simulink model "mBraccioSimulation"  (R2021a)
settings: Solver=VariableStepAuto  StartTime=0.0  StopTime=inf  RelTol=1e-3
undefined symbols (not defined in the file): adHomeConfig, adMotorLimits, adWaypoints, adWeight, Levenberg, Marquardt
libraries: vrlib x3, robotcorelib x2, robotmaniplib x2
settings Model: Creator=angelo  LastModifiedBy=angelo

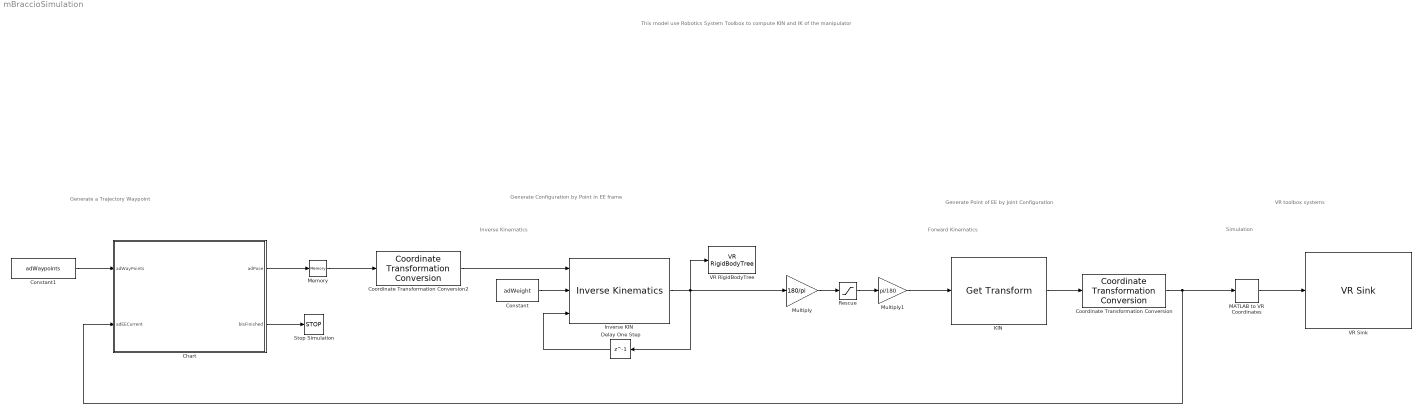
== system mBraccioSimulation ==
  note: Generate a Trajectory Waypoint
  note: Generate Point of EE by Joint Configuration
  note: Forward Kinematics
  note: Inverse Kinematics
  note: Simulation
  note: This model use Robotics System Toolbox to compute KIN and IK of the manipulator
  note: Generate Configuration by Point in EE frame
  note: VR toolbox systems
  Chart : Stateflow chart  TreatAsAtomicUnit=on
  Constant : Constant  Value=adWeight
  Constant1 : Constant  Value=adWaypoints
  Coordinate Transformation Conversion : robotcorelib/Coordinate Transformation Conversion  InputRepresentation=Homogeneous Transformation  InputEulerSequence=ZYX  ShowTrVecInputPort=on  OutputRepresentation=Translation Vector  OutputEulerSequence=ZYX  ShowTrVecOutputPort=on  SimulateUsing=Interpreted execution
      settings: SourceProductBaseCode=NV,RO,RR,UV
  Coordinate Transformation Conversion2 : robotcorelib/Coordinate Transformation Conversion  InputRepresentation=Translation Vector  InputEulerSequence=ZYX  ShowTrVecInputPort=on  OutputRepresentation=Homogeneous Transformation  OutputEulerSequence=ZYX  ShowTrVecOutputPort=on  SimulateUsing=Interpreted execution
      settings: SourceProductBaseCode=NV,RO,RR,UV
  Delay One Step : Delay  DelayLength=1  InitialCondition=adHomeConfig
  Inverse KIN : robotmaniplib/Inverse Kinematics  RigidBodyTree=oRbtBraccio  EndEffector=ee  ShowInfo=off  SolverName=Levenberg-Marquardt  EnforceJointLimits=on  MaxIterations=1500  MaxTime=10  GradientTolerance=1e-7  SolutionTolerance=1e-6  StepTolerance=1e-14  ErrorChangeTolerance=1e-12  UseErrorDamping=on  DampingBias=0.0025  SimulateUsing=Interpreted execution
  KIN : robotmaniplib/Get Transform  RigidBodyTree=oRbtBraccio  SourceBody=ee  TargetBody=base_link  SimulateUsing=Interpreted execution
  MATLAB to VR Coordinates : vrlib/Utilities/MATLAB to VR Coordinates
      settings: SourceProductBaseCode=SL
  Memory : Memory
  Multiply : Gain  Gain=180/pi
  Multiply1 : Gain  Gain=pi/180
  Rescue : Saturate  UpperLimit=adMotorLimits(:,2)  LowerLimit=adMotorLimits(:,1)
  Stop Simulation : Stop
  VR RigidBodyTree : vrlib/VR RigidBodyTree  VrmlFile=/home/angelo/1.PROJECTS/arm-manipulator-6dof/graphics/robotWorld.x3d  RBT=oRbtBraccio  useRBT=off  Ts=-1  ForceViewerOpen=off
      settings: SourceProductBaseCode=SL
  VR Sink : vrlib/VR Sink  InstantiateOnLoad=on  SampleTime=0.1  ViewEnable=on  RemoteChange=off  RemoteView=off  FieldsWritten=SetPoint.translation.3.1.1.double  WorldFileName=graphics/robotWorld.x3d  AutoView=on  VideoDimensions=[]  AllowVariableSize=off
  wires:
  Delay One Step/1 -> Inverse KIN/3
  Inverse KIN/1 -> VR RigidBodyTree/1, Multiply/1, Delay One Step/1
  KIN/1 -> Coordinate Transformation Conversion/1
  MATLAB to VR Coordinates/1 -> VR Sink/1
  Coordinate Transformation Conversion/1 -> MATLAB to VR Coordinates/1, Chart/2(adEECurrent)
  Constant/1 -> Inverse KIN/2
  Multiply/1 -> Rescue/1
  Rescue/1 -> Multiply1/1
  Multiply1/1 -> KIN/1
  Coordinate Transformation Conversion2/1 -> Inverse KIN/1
  Chart/2(bIsFinished) -> Stop Simulation/1
  Chart/1(adPose) -> Memory/1
  Memory/1 -> Coordinate Transformation Conversion2/1
  Constant1/1 -> Chart/1(adWayPoints)

== stateflow chart mBraccioSimulation/Chart ==
  settings: executeAtInitialization=1
  (default) -> (junction 3) : {adError = vecnorm((adPose - adEECurrent), 2, 1);}
  (junction 3) -> (junction 7) [order 1] : [all(adError < tol)]
  (junction 7) -> (junction 11) [order 1] : [i == length(adWayPoints)]
  (junction 3) -> (junction 22) [order 2]
  (junction 7) -> (junction 17) [order 2] : {i = i + 1;}
  (junction 11) -> (junction 14) : {bIsFinished = true;}
  (junction 17) -> (junction 22)
  (junction 14) -> (junction 17)
  (junction 22) -> (junction 26) : { adPose = adWayPoints(:, i) ; }
  data: adWayPoints input; adEECurrent input; adError local; tol local =.01; adPose output =adStartPoint'; bIsFinished output =false; i local =1
